simulink model "afm_z_simple"  (R2018a)
settings: Solver=VariableStepAuto  StartTime=0.0  StopTime=trun  RelTol=1e-3
libraries: cstblocks x4
settings Model: Creator=arnold  LastModifiedBy=arnold

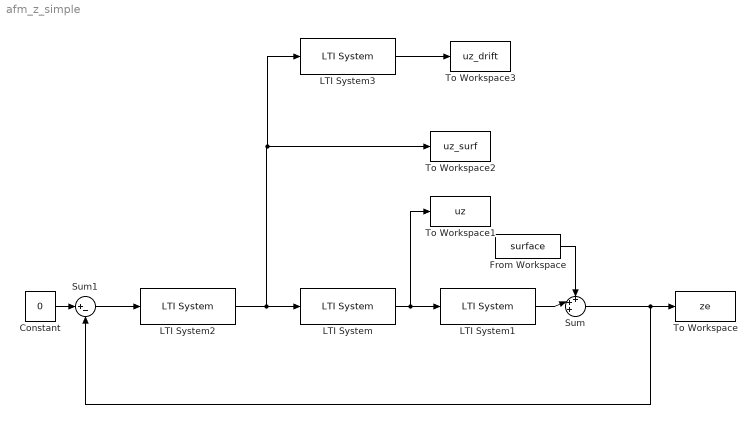
== system afm_z_simple ==
  Constant : Constant  Value=0
  From Workspace : FromWorkspace  VariableName=surface  SampleTime=0
  LTI System : cstblocks/LTI System  sys=Dz  IC=[]
  LTI System1 : cstblocks/LTI System  sys=G_plant  IC=[]
  LTI System2 : cstblocks/LTI System  sys=D_I  IC=[]
  LTI System3 : cstblocks/LTI System  sys=gdrift  IC=[]
  Sum : Sum  Inputs=+++|
  Sum1 : Sum  Inputs=|+-
  To Workspace : ToWorkspace  VariableName=ze  SaveFormat=Timeseries  SampleTime=-1
  To Workspace1 : ToWorkspace  VariableName=uz  SaveFormat=Timeseries  SampleTime=-1
  To Workspace2 : ToWorkspace  VariableName=uz_surf  SaveFormat=Timeseries  SampleTime=-1
  To Workspace3 : ToWorkspace  VariableName=uz_drift  SaveFormat=Timeseries  SampleTime=-1
  wires:
  From Workspace/1 -> Sum/1
  Sum1/1 -> LTI System2/1
  Constant/1 -> Sum1/1
  LTI System/1 -> To Workspace1/1, LTI System1/1
  LTI System1/1 -> Sum/2
  Sum/1 -> To Workspace/1, Sum1/2
  LTI System2/1 -> LTI System3/1, To Workspace2/1, LTI System/1
  LTI System3/1 -> To Workspace3/1
